simulink model "planta"  (Simulink 7.3)
settings: Solver=ode45  StartTime=0.0  StopTime=2.5  RelTol=1e-3
settings Model: Creator=Luis Diaz  LastModifiedBy=Luis Diaz

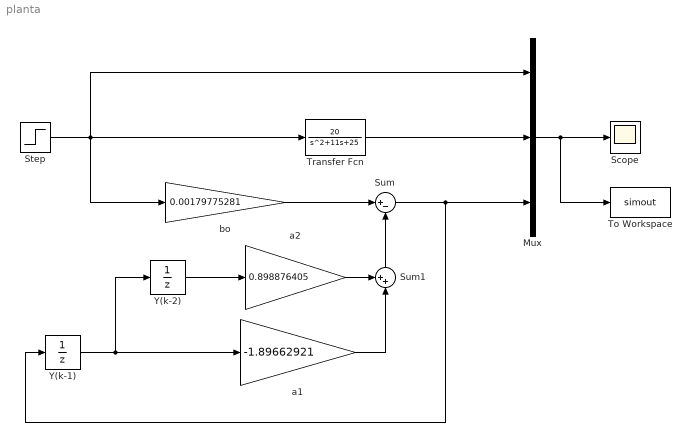
== system planta ==
  Mux : Mux  Inputs=3
  Scope : Scope
  Step : Step  Time=0.1  SampleTime=0
  Sum : Sum  Inputs=|+-  OutDataType=fixdt(1, 16)  OutScaling=2^0
  Sum1 : Sum  Inputs=++|  OutDataType=fixdt(1, 16)  OutScaling=2^0
  To Workspace : ToWorkspace  VariableName=simout  SampleTime=-1  SaveFormat=Structure
  Transfer Fcn : TransferFcn  Numerator=[20]  Denominator=[1 11 25]
  Y(k-1) : UnitDelay  SampleTime=0.01
  Y(k-2) : UnitDelay  SampleTime=0.01
  a1 : Gain  Gain=-1.89662921  ParameterDataType=fixdt(1, 16)  ParameterScaling=2^0  OutDataType=fixdt(1, 16)  OutScaling=2^0
  a2 : Gain  Gain=0.898876405  ParameterDataType=fixdt(1, 16)  ParameterScaling=2^0  OutDataType=fixdt(1, 16)  OutScaling=2^0
  bo : Gain  Gain=0.00179775281  ParameterDataType=fixdt(1, 16)  ParameterScaling=2^0  OutDataType=fixdt(1, 16)  OutScaling=2^0
  wires:
  Mux/1 -> Scope/1, To Workspace/1
  Transfer Fcn/1 -> Mux/2
  bo/1 -> Sum/1
  Sum/1 -> Y(k-1)/1, Mux/3
  Y(k-1)/1 -> Y(k-2)/1, a1/1
  Y(k-2)/1 -> a2/1
  a1/1 -> Sum1/2
  a2/1 -> Sum1/1
  Sum1/1 -> Sum/2
  Step/1 -> Transfer Fcn/1, Mux/1, bo/1
